simulink model "pract_2"  (R2020b)
settings: Solver=VariableStepAuto  StartTime=0.0  StopTime=10.0  RelTol=1e-3
libraries: commutil2 x2, dspquant2 x2
settings Model: Creator=Egor  LastModifiedBy=Egor

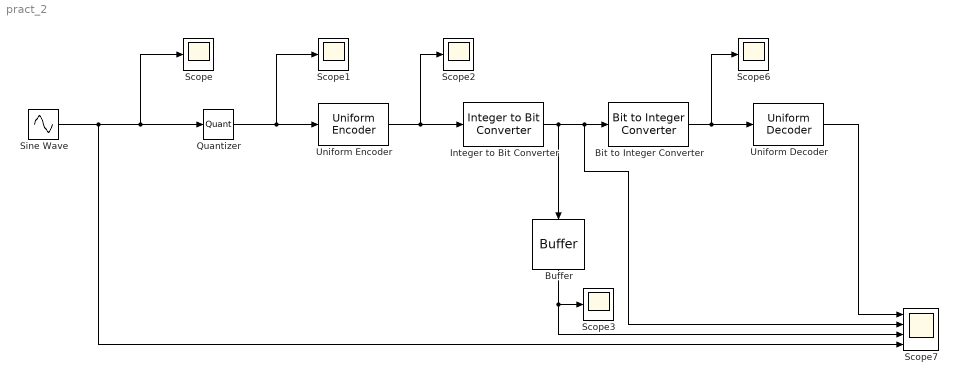
== system pract_2 ==
  Bit to Integer Converter : commutil2/Bit to Integer Converter  nbits=8  bitOrder=MSB first  signedOutputValues=Unsigned  outDtype=Inherit via internal rule  outDtypeSigned=Inherit via internal rule
  Buffer : Buffer  N=1  OutputFrames=off
  Integer to Bit Converter : commutil2/Integer to Bit Converter  nbits=8  signedInputValues=Unsigned  bitOrder=MSB first  outDtype=Inherit via internal rule
  Quantizer : Quantizer  QuantizationInterval=0.7
  Scope{,1..3,6} (5 alike) : Scope
  Scope7 : Scope  NumInputPorts=4
  Sine Wave : Sin  Amplitude=5.5  Frequency=314.16  Phase=1.745  SampleTime=0.0001
  Uniform Decoder : dspquant2/Uniform Decoder  peak=5.5  bits=8  overflowMode=Saturate  otype=Double
      settings: SourceProductBaseCode=DS
  Uniform Encoder : dspquant2/Uniform Encoder  peak=5.5  bits=8  otype=Unsigned integer
  wires:
  Sine Wave/1 -> Scope7/4, Quantizer/1, Scope/1
  Quantizer/1 -> Uniform Encoder/1, Scope1/1
  Uniform Encoder/1 -> Integer to Bit Converter/1, Scope2/1
  Bit to Integer Converter/1 -> Uniform Decoder/1, Scope6/1
  Uniform Decoder/1 -> Scope7/1
  Buffer/1 -> Scope7/3, Scope3/1
  Integer to Bit Converter/1 -> Scope7/2, Bit to Integer Converter/1, Buffer/1
